simulink library "halout"  (R2021b)
settings: Solver=VariableStepAuto  StartTime=0.0  StopTime=10.0  RelTol=1e-3
undefined symbols (not defined in the file): C_TASK_5MS_S, FALSE, KHAL_CAN1FD1APS3E2E_flg, KHAL_CAN1FD1APS3TxReq_flg, KHAL_CAN1FD1VCU2E2E_flg, KHAL_CAN1FD1VCU2TxReq_flg, KHAL_CAN1FD1VCU3E2E_flg, KHAL_CAN1FD1VCU3TxReq_flg, KHAL_CAN1TxReq_flg, KHAL_CAN1VMCFCM1E2E_flg, KHAL_CAN1VMCFCM1TxReq_flg, KHAL_CAN2TxReq_flg, KHAL_CAN3FD3VCU1toNIDECTxReq_flg, KHAL_CAN3FD3VCU1TxReq_flg, KHAL_CAN3FD3VCU2E2E_flg, KHAL_CAN3FD3VCU2toNIDECE2E_flg, KHAL_CAN3FD3VCU2toNIDECTxReq_flg, KHAL_CAN3FD3VCU2TxReq_flg, KHAL_CAN3TxReq_flg, KHAL_CAN4FD4CE1000E2E_flg, KHAL_CAN4FD4CE1000TxReq_flg, KHAL_CAN4TxReq_flg, KHAL_CAN5TxReq_flg, KHAL_CAN6FD6APS3E2E_flg, KHAL_CAN6FD6APS3TxReq_flg, KHAL_CAN6FD6VCU2E2E_flg, KHAL_CAN6FD6VCU2TxReq_flg, KHAL_CAN6TxReq_flg, ONE_INT, TRUE, ZERO_INT
libraries: FVT_lib x549, simulink x244
(part 12 of 27)

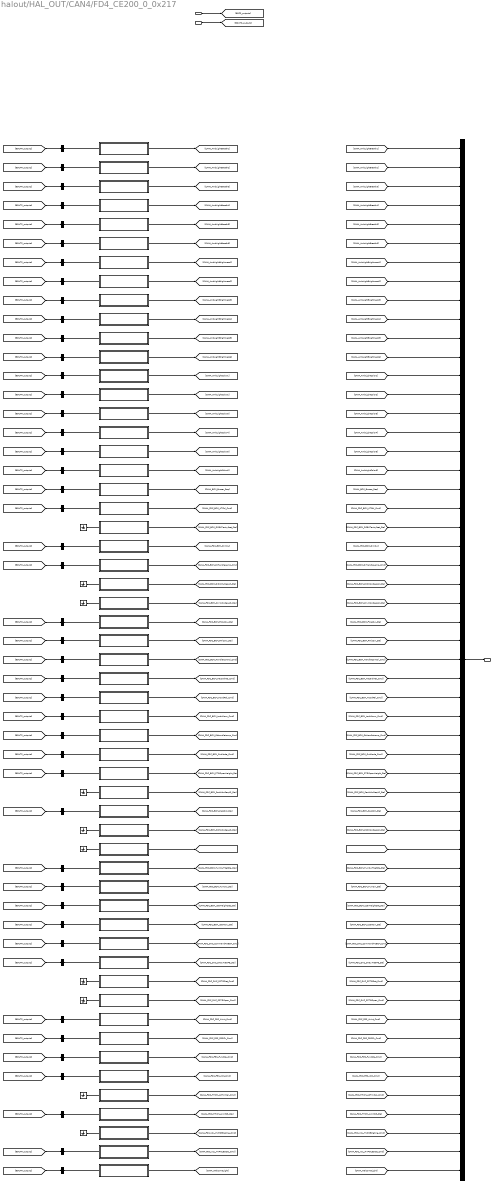
== system halout/HAL_OUT/CAN4/FD4_CE200_0_0x217 ==
  BSCP_outputs : Inport  OutDataTypeStr=Bus: BSCP_outputs
  BOUTP_outputs : Inport  Port=2  OutDataTypeStr=Bus: BOUTP_outputs
  AmbLightBreath1 : Subsystem
  AmbLightBreath2 : Subsystem
  AmbLightBreath3 : Subsystem
  AmbLightBreath4 : Subsystem
  AmbLightBreath5 : Subsystem
  AmbLightBreath6 : Subsystem
  AmbLightBrightness1 : Subsystem
  AmbLightBrightness2 : Subsystem
  AmbLightBrightness3 : Subsystem
  AmbLightBrightness4 : Subsystem
  AmbLightBrightness5 : Subsystem
  AmbLightBrightness6 : Subsystem
  AmbLightColor1 : Subsystem
  AmbLightColor2 : Subsystem
  AmbLightColor3 : Subsystem
  AmbLightColor4 : Subsystem
  AmbLightColor5 : Subsystem
  AmbLightColor6 : Subsystem
  BCMBuzzerReq : Subsystem
  FDCBCMATCtrlCmd : Subsystem
  FDCBCMDSEATentryfsetSta : Subsystem
  FDCBCMDimSw : Subsystem
  FDCBCMDrHandleLampCmd : Subsystem
  FDCBCMDrRWdwReqAPSta : Subsystem
  FDCBCMDrvWdwReqAPSta : Subsystem
  FDCBCMFWasSwSta : Subsystem
  FDCBCMFWipSwSta : Subsystem
  FDCBCMHandleControlCmd : Subsystem
  FDCBCMHazardINDCmd : Subsystem
  FDCBCMHoodRelCmd : Subsystem
  FDCBCMLockAlarmCmd : Subsystem
  FDCBCMOtHandleLampCmd : Subsystem
  FDCBCMOutModeCmd : Subsystem
  FDCBCMPTGOpenHeightSta : Subsystem
  FDCBCMPasWdwReqAPSta : Subsystem
  FDCBCMPassSWSta : Subsystem
  FDCBCMPsRWdwReqAPSta : Subsystem
  FDCBCMSettingUpdateReqCmd : Subsystem
  FDCBCMTurnSwSta : Subsystem
  FDCBCMTurnSwTSetStaSta : Subsystem
  FDCBCMUserHeightSetSta : Subsystem
  FDCBCMUserNowSta : Subsystem
  FDCDKCCommandToBCMCmd : Subsystem
  FDCDKCDKeyAreaPESta : Subsystem
  FDCDKCSPTGDetCmd : Subsystem
  FDCDKCSPTGOpenCmd : Subsystem
  FDCFGSAirIntCmd : Subsystem
  FDCFGSFGSChCmd : Subsystem
  FDCFGSFuncStaCmd : Subsystem
  FDCFGSIONCmd : Subsystem
  FDCTHCMACTInitialCmd : Subsystem
  FDCTHCMAirIntZ3Sta : Subsystem
  FDCV2LHVPOBklgtingCmd : Subsystem
  FDCV2LHVPOLEDStsCmd : Subsystem
  Ground{,2..3,6..12} (10 alike) : Ground
  WelcomeLight : Subsystem
  bus_creator : BusCreator  Inputs=55  OutDataTypeStr=Bus: DT_CAN4_SG_FD4_CE200_0  NonVirtualBus=on
  bus_selector : BusSelector  OutputSignals=VOUTP_AmbLightBreath1_enum
  bus_selector1 : BusSelector  OutputSignals=VOUTP_AmbLightBreath2_enum
  bus_selector10 : BusSelector  OutputSignals=VOUTP_AmbLightBrightness5_enum
  bus_selector11 : BusSelector  OutputSignals=VOUTP_AmbLightBrightness6_enum
  bus_selector12 : BusSelector  OutputSignals=VOUTP_AmbLightColor1_enum
  bus_selector13 : BusSelector  OutputSignals=VOUTP_AmbLightColor2_enum
  bus_selector14 : BusSelector  OutputSignals=VOUTP_AmbLightColor3_enum
  bus_selector15 : BusSelector  OutputSignals=VOUTP_AmbLightColor4_enum
  bus_selector16 : BusSelector  OutputSignals=VOUTP_AmbLightColor5_enum
  bus_selector17 : BusSelector  OutputSignals=VOUTP_AmbLightColor6_enum
  bus_selector18 : BusSelector  OutputSignals=VOUTP_BCMBuzzerReq_flg
  bus_selector19 : BusSelector  OutputSignals=VOUTP_ATCtrl_enum
  bus_selector2 : BusSelector  OutputSignals=VOUTP_AmbLightBreath3_enum
  bus_selector20 : BusSelector  OutputSignals=VOUTP_DimSwSta_flg
  bus_selector21 : BusSelector  OutputSignals=VOUTP_FWasSwSta_enum
  bus_selector22 : BusSelector  OutputSignals=VOUTP_FWipSwSta_enum
  bus_selector23 : BusSelector  OutputSignals=VOUTP_HazardIND_flg
  bus_selector24 : BusSelector  OutputSignals=VOUTP_HoodRelCmd_flg
  bus_selector25 : BusSelector  OutputSignals=VOUTP_LockAlarm_enum
  bus_selector26 : BusSelector  OutputSignals=VOUTP_OutMode_enum
  bus_selector27 : BusSelector  OutputSignals=VOUTP_PTGOpenHeightSta_enum
  bus_selector28 : BusSelector  OutputSignals=VOUTP_PassSWSta_flg
  bus_selector29 : BusSelector  OutputSignals=VOUTP_TurnSwTSetSta_enum
  bus_selector3 : BusSelector  OutputSignals=VOUTP_AmbLightBreath4_enum
  bus_selector30 : BusSelector  OutputSignals=VOUTP_TurnSwSta_enum
  bus_selector31 : BusSelector  OutputSignals=VOUTP_UserHeightSet_cnt
  bus_selector32 : BusSelector  OutputSignals=VOUTP_UserNow_enum
  bus_selector33 : BusSelector  OutputSignals=VOUTP_PCommandToBCM_enum
  bus_selector34 : BusSelector  OutputSignals=VOUTP_KeyAreaLockUnlock_enum
  bus_selector35 : BusSelector  OutputSignals=VOUTP_FDCFGSAirIntCmd_enum
  bus_selector36 : BusSelector  OutputSignals=VOUTP_FDCFGSChCmd_enum
  bus_selector37 : BusSelector  OutputSignals=VOUTP_FDCFGSFuncSta_flg
  bus_selector38 : BusSelector  OutputSignals=VOUTP_FDCFGSIONCmd_flg
  bus_selector39 : BusSelector  OutputSignals=VOUTP_FDCTHCAirIntZ3Sta_enum
  bus_selector4 : BusSelector  OutputSignals=VOUTP_AmbLightBreath5_enum
  bus_selector40 : BusSelector  OutputSignals=VOUTP_HVPO120VGrpALDSt_enum
  bus_selector41 : BusSelector  OutputSignals=VOUTP_WelcomeLight_enum
  bus_selector42 : BusSelector  OutputSignals=VOUTP_FDLHandleLampCmd_flg
  bus_selector43 : BusSelector  OutputSignals=VOUTP_FDHandleCmd_enum
  bus_selector44 : BusSelector  OutputSignals=VOUTP_FDRHandleLampCmd_flg
  bus_selector5 : BusSelector  OutputSignals=VOUTP_AmbLightBreath6_enum
  bus_selector6 : BusSelector  OutputSignals=VOUTP_AmbLightBrightness1_enum
  bus_selector7 : BusSelector  OutputSignals=VOUTP_AmbLightBrightness2_enum
  bus_selector8 : BusSelector  OutputSignals=VOUTP_AmbLightBrightness3_enum
  bus_selector9 : BusSelector  OutputSignals=VOUTP_AmbLightBrightness4_enum
  FD4_CE200_0 : Outport
  wires:
  BSCP_outputs/1 -> [BSCP_outputs]
  BOUTP_outputs/1 -> [BOUTP_outputs]
  [CAN4_AmbLightBreath1] -> bus_creator/1  "CAN4_AmbLightBreath1"
  [CAN4_AmbLightBreath2] -> bus_creator/2  "CAN4_AmbLightBreath2"
  [CAN4_AmbLightBreath3] -> bus_creator/3  "CAN4_AmbLightBreath3"
  [CAN4_AmbLightBreath4] -> bus_creator/4  "CAN4_AmbLightBreath4"
  [CAN4_AmbLightBreath5] -> bus_creator/5  "CAN4_AmbLightBreath5"
  [CAN4_AmbLightBreath6] -> bus_creator/6  "CAN4_AmbLightBreath6"
  [CAN4_AmbLightBrightness1] -> bus_creator/7  "CAN4_AmbLightBrightness1"
  [CAN4_AmbLightBrightness2] -> bus_creator/8  "CAN4_AmbLightBrightness2"
  [CAN4_AmbLightBrightness3] -> bus_creator/9  "CAN4_AmbLightBrightness3"
  [CAN4_AmbLightBrightness4] -> bus_creator/10  "CAN4_AmbLightBrightness4"
  [CAN4_AmbLightBrightness5] -> bus_creator/11  "CAN4_AmbLightBrightness5"
  [CAN4_AmbLightBrightness6] -> bus_creator/12  "CAN4_AmbLightBrightness6"
  [CAN4_AmbLightColor1] -> bus_creator/13  "CAN4_AmbLightColor1"
  [CAN4_AmbLightColor2] -> bus_creator/14  "CAN4_AmbLightColor2"
  [CAN4_AmbLightColor3] -> bus_creator/15  "CAN4_AmbLightColor3"
  [CAN4_AmbLightColor4] -> bus_creator/16  "CAN4_AmbLightColor4"
  [CAN4_AmbLightColor5] -> bus_creator/17  "CAN4_AmbLightColor5"
  [CAN4_AmbLightColor6] -> bus_creator/18  "CAN4_AmbLightColor6"
  [CAN4_BCM_Buzzer_Req] -> bus_creator/19  "CAN4_BCM_Buzzer_Req"
  [CAN4_FDC_BCM_ATCtrl_Cmd] -> bus_creator/20  "CAN4_FDC_BCM_ATCtrl_Cmd"
  [CAN4_FDC_BCM_DSEATentryfset_Sta] -> bus_creator/21  "CAN4_FDC_BCM_DSEATentryfset_Sta"
  [CAN4_FDC_BCM_DimSw] -> bus_creator/22  "CAN4_FDC_BCM_DimSw"
  [CAN4_FDC_BCM_DrHandleLamp_Cmd] -> bus_creator/23  "CAN4_FDC_BCM_DrHandleLamp_Cmd"
  [CAN4_FDC_BCM_DrRWdwReqAP_Sta] -> bus_creator/24  "CAN4_FDC_BCM_DrRWdwReqAP_Sta"
  [CAN4_FDC_BCM_DrvWdwReqAP_Sta] -> bus_creator/25  "CAN4_FDC_BCM_DrvWdwReqAP_Sta"
  [CAN4_FDC_BCM_FWasSw_Sta] -> bus_creator/26  "CAN4_FDC_BCM_FWasSw_Sta"
  [CAN4_FDC_BCM_FWipSw_Sta] -> bus_creator/27  "CAN4_FDC_BCM_FWipSw_Sta"
  [CAN4_FDC_BCM_HandleControl_Cmd] -> bus_creator/28  "CAN4_FDC_BCM_HandleControl_Cmd"
  [CAN4_FDC_BCM_HazardIND_Cmd] -> bus_creator/29  "CAN4_FDC_BCM_HazardIND_Cmd"
  [CAN4_FDC_BCM_HoodRel_Cmd] -> bus_creator/30  "CAN4_FDC_BCM_HoodRel_Cmd"
  [CAN4_FDC_BCM_LockAlarm_Cmd] -> bus_creator/31  "CAN4_FDC_BCM_LockAlarm_Cmd"
  [CAN4_FDC_BCM_OtHandleLamp_Cmd] -> bus_creator/32  "CAN4_FDC_BCM_OtHandleLamp_Cmd"
  [CAN4_FDC_BCM_OutMode_Cmd] -> bus_creator/33  "CAN4_FDC_BCM_OutMode_Cmd"
  [CAN4_FDC_BCM_PTGOpenHeight_Sta] -> bus_creator/34  "CAN4_FDC_BCM_PTGOpenHeight_Sta"
  [CAN4_FDC_BCM_PasWdwReqAP_Sta] -> bus_creator/35  "CAN4_FDC_BCM_PasWdwReqAP_Sta"
  [CAN4_FDC_BCM_PassSW_Sta] -> bus_creator/36  "CAN4_FDC_BCM_PassSW_Sta"
  [CAN4_FDC_BCM_PsRWdwReqAP_Sta] -> bus_creator/37  "CAN4_FDC_BCM_PsRWdwReqAP_Sta"
  [CAN4_FDC_BCM_SettingUpdateReq_Cmd] -> bus_creator/38  "CAN4_FDC_BCM_SettingUpdateReq_Cmd"
  [CAN4_FDC_BCM_TurnSwTSetSta_Sta] -> bus_creator/39  "CAN4_FDC_BCM_TurnSwTSetSta_Sta"
  [CAN4_FDC_BCM_TurnSw_Sta] -> bus_creator/40  "CAN4_FDC_BCM_TurnSw_Sta"
  [CAN4_FDC_BCM_UserHeightSet_Sta] -> bus_creator/41  "CAN4_FDC_BCM_UserHeightSet_Sta"
  [CAN4_FDC_BCM_UserNow_Sta] -> bus_creator/42  "CAN4_FDC_BCM_UserNow_Sta"
  [CAN4_FDC_DKC_CommandToBCM_Cmd] -> bus_creator/43  "CAN4_FDC_DKC_CommandToBCM_Cmd"
  [CAN4_FDC_DKC_DKeyAreaPE_Sta] -> bus_creator/44  "CAN4_FDC_DKC_DKeyAreaPE_Sta"
  [CAN4_FDC_DKC_SPTGDet_Cmd] -> bus_creator/45  "CAN4_FDC_DKC_SPTGDet_Cmd"
  [CAN4_FDC_DKC_SPTGOpen_Cmd] -> bus_creator/46  "CAN4_FDC_DKC_SPTGOpen_Cmd"
  [CAN4_FDC_FGS_AirInt_Cmd] -> bus_creator/47  "CAN4_FDC_FGS_AirInt_Cmd"
  [CAN4_FDC_FGS_FGSCh_Cmd] -> bus_creator/48  "CAN4_FDC_FGS_FGSCh_Cmd"
  [CAN4_FDC_FGS_FuncSta_Cmd] -> bus_creator/49  "CAN4_FDC_FGS_FuncSta_Cmd"
  [CAN4_FDC_FGS_ION_Cmd] -> bus_creator/50  "CAN4_FDC_FGS_ION_Cmd"
  [CAN4_FDC_THCM_ACTInitial_Cmd] -> bus_creator/51  "CAN4_FDC_THCM_ACTInitial_Cmd"
  [CAN4_FDC_THCM_AirIntZ3_Sta] -> bus_creator/52  "CAN4_FDC_THCM_AirIntZ3_Sta"
  [CAN4_FDC_V2L_HVPOBklgting_Cmd] -> bus_creator/53  "CAN4_FDC_V2L_HVPOBklgting_Cmd"
  [CAN4_FDC_V2L_HVPOLEDSts_Cmd] -> bus_creator/54  "CAN4_FDC_V2L_HVPOLEDSts_Cmd"
  [CAN4_WelcomeLight] -> bus_creator/55  "CAN4_WelcomeLight"
  bus_creator/1 -> FD4_CE200_0/1
  AmbLightBreath1/1(CAN4_AmbLightBreath1) -> [CAN4_AmbLightBreath1]
  AmbLightBreath2/1(CAN4_AmbLightBreath2) -> [CAN4_AmbLightBreath2]
  AmbLightBreath3/1(CAN4_AmbLightBreath3) -> [CAN4_AmbLightBreath3]
  AmbLightBreath4/1(CAN4_AmbLightBreath4) -> [CAN4_AmbLightBreath4]
  AmbLightBreath5/1(CAN4_AmbLightBreath5) -> [CAN4_AmbLightBreath5]
  AmbLightBreath6/1(CAN4_AmbLightBreath6) -> [CAN4_AmbLightBreath6]
  AmbLightBrightness1/1(CAN4_AmbLightBrightness1) -> [CAN4_AmbLightBrightness1]
  AmbLightBrightness2/1(CAN4_AmbLightBrightness2) -> [CAN4_AmbLightBrightness2]
  AmbLightBrightness3/1(CAN4_AmbLightBrightness3) -> [CAN4_AmbLightBrightness3]
  AmbLightBrightness4/1(CAN4_AmbLightBrightness4) -> [CAN4_AmbLightBrightness4]
  AmbLightBrightness5/1(CAN4_AmbLightBrightness5) -> [CAN4_AmbLightBrightness5]
  AmbLightBrightness6/1(CAN4_AmbLightBrightness6) -> [CAN4_AmbLightBrightness6]
  AmbLightColor1/1(CAN4_AmbLightColor1) -> [CAN4_AmbLightColor1]
  AmbLightColor2/1(CAN4_AmbLightColor2) -> [CAN4_AmbLightColor2]
  AmbLightColor3/1(CAN4_AmbLightColor3) -> [CAN4_AmbLightColor3]
  AmbLightColor4/1(CAN4_AmbLightColor4) -> [CAN4_AmbLightColor4]
  AmbLightColor5/1(CAN4_AmbLightColor5) -> [CAN4_AmbLightColor5]
  AmbLightColor6/1(CAN4_AmbLightColor6) -> [CAN4_AmbLightColor6]
  BCMBuzzerReq/1(CAN4_BCM_Buzzer_Req) -> [CAN4_BCM_Buzzer_Req]
  FDCBCMATCtrlCmd/1(CAN4_FDC_BCM_ATCtrl_Cmd) -> [CAN4_FDC_BCM_ATCtrl_Cmd]
  FDCBCMDSEATentryfsetSta/1(CAN4_FDC_BCM_DSEATentryfset_Sta) -> [CAN4_FDC_BCM_DSEATentryfset_Sta]
  FDCBCMDimSw/1(CAN4_FDC_BCM_DimSw) -> [CAN4_FDC_BCM_DimSw]
  FDCBCMDrHandleLampCmd/1(CAN4_FDC_BCM_DrHandleLamp_Cmd) -> [CAN4_FDC_BCM_DrHandleLamp_Cmd]
  FDCBCMDrRWdwReqAPSta/1(CAN4_FDC_BCM_DrRWdwReqAP_Sta) -> [CAN4_FDC_BCM_DrRWdwReqAP_Sta]
  FDCBCMDrvWdwReqAPSta/1(CAN4_FDC_BCM_DrvWdwReqAP_Sta) -> [CAN4_FDC_BCM_DrvWdwReqAP_Sta]
  FDCBCMFWasSwSta/1(CAN4_FDC_BCM_FWasSw_Sta) -> [CAN4_FDC_BCM_FWasSw_Sta]
  FDCBCMFWipSwSta/1(CAN4_FDC_BCM_FWipSw_Sta) -> [CAN4_FDC_BCM_FWipSw_Sta]
  FDCBCMHandleControlCmd/1(CAN4_FDC_BCM_HandleControl_Cmd) -> [CAN4_FDC_BCM_HandleControl_Cmd]
  FDCBCMHazardINDCmd/1(CAN4_FDC_BCM_HazardIND_Cmd) -> [CAN4_FDC_BCM_HazardIND_Cmd]
  FDCBCMHoodRelCmd/1(CAN4_FDC_BCM_HoodRel_Cmd) -> [CAN4_FDC_BCM_HoodRel_Cmd]
  FDCBCMLockAlarmCmd/1(CAN4_FDC_BCM_LockAlarm_Cmd) -> [CAN4_FDC_BCM_LockAlarm_Cmd]
  FDCBCMOtHandleLampCmd/1(CAN4_FDC_BCM_OtHandleLamp_Cmd) -> [CAN4_FDC_BCM_OtHandleLamp_Cmd]
  FDCBCMOutModeCmd/1(CAN4_FDC_BCM_OutMode_Cmd) -> [CAN4_FDC_BCM_OutMode_Cmd]
  FDCBCMPTGOpenHeightSta/1(CAN4_FDC_BCM_PTGOpenHeight_Sta) -> [CAN4_FDC_BCM_PTGOpenHeight_Sta]
  FDCBCMPasWdwReqAPSta/1(CAN4_FDC_BCM_PasWdwReqAP_Sta) -> [CAN4_FDC_BCM_PasWdwReqAP_Sta]
  FDCBCMPassSWSta/1(CAN4_FDC_BCM_PassSW_Sta) -> [CAN4_FDC_BCM_PassSW_Sta]
  FDCBCMPsRWdwReqAPSta/1(CAN4_FDC_BCM_PsRWdwReqAP_Sta) -> [CAN4_FDC_BCM_PsRWdwReqAP_Sta]
  FDCBCMSettingUpdateReqCmd/1(CAN4_FDC_BCM_SettingUpdateReq_Cmd) -> [CAN4_FDC_BCM_SettingUpdateReq_Cmd]
  FDCBCMTurnSwTSetStaSta/1(CAN4_FDC_BCM_TurnSwTSetSta_Sta) -> [CAN4_FDC_BCM_TurnSwTSetSta_Sta]
  FDCBCMTurnSwSta/1(CAN4_FDC_BCM_TurnSw_Sta) -> [CAN4_FDC_BCM_TurnSw_Sta]
  FDCBCMUserHeightSetSta/1(CAN4_FDC_BCM_UserHeightSet_Sta) -> [CAN4_FDC_BCM_UserHeightSet_Sta]
  FDCBCMUserNowSta/1(CAN4_FDC_BCM_UserNow_Sta) -> [CAN4_FDC_BCM_UserNow_Sta]
  FDCDKCCommandToBCMCmd/1(CAN4_FDC_DKC_CommandToBCM_Cmd) -> [CAN4_FDC_DKC_CommandToBCM_Cmd]
  FDCDKCDKeyAreaPESta/1(CAN4_FDC_DKC_DKeyAreaPE_Sta) -> [CAN4_FDC_DKC_DKeyAreaPE_Sta]
  FDCDKCSPTGDetCmd/1(CAN4_FDC_DKC_SPTGDet_Cmd) -> [CAN4_FDC_DKC_SPTGDet_Cmd]
  FDCDKCSPTGOpenCmd/1(CAN4_FDC_DKC_SPTGOpen_Cmd) -> [CAN4_FDC_DKC_SPTGOpen_Cmd]
  FDCFGSAirIntCmd/1(CAN4_FDC_FGS_AirInt_Cmd) -> [CAN4_FDC_FGS_AirInt_Cmd]
  FDCFGSFGSChCmd/1(CAN4_FDC_FGS_FGSCh_Cmd) -> [CAN4_FDC_FGS_FGSCh_Cmd]
  FDCFGSFuncStaCmd/1(CAN4_FDC_FGS_FuncSta_Cmd) -> [CAN4_FDC_FGS_FuncSta_Cmd]
  FDCFGSIONCmd/1(CAN4_FDC_FGS_ION_Cmd) -> [CAN4_FDC_FGS_ION_Cmd]
  FDCTHCMACTInitialCmd/1(CAN4_FDC_THCM_ACTInitial_Cmd) -> [CAN4_FDC_THCM_ACTInitial_Cmd]
  FDCTHCMAirIntZ3Sta/1(CAN4_FDC_THCM_AirIntZ3_Sta) -> [CAN4_FDC_THCM_AirIntZ3_Sta]
  FDCV2LHVPOBklgtingCmd/1(CAN4_FDC_V2L_HVPOBklgting_Cmd) -> [CAN4_FDC_V2L_HVPOBklgting_Cmd]
  FDCV2LHVPOLEDStsCmd/1(CAN4_FDC_V2L_HVPOLEDSts_Cmd) -> [CAN4_FDC_V2L_HVPOLEDSts_Cmd]
  WelcomeLight/1(CAN4_WelcomeLight) -> [CAN4_WelcomeLight]
  bus_selector/1 -> AmbLightBreath1/1(AmbLightBreath1)  "<VOUTP_AmbLightBreath1_enum>"
  [BOUTP_outputs] -> bus_selector/1
  bus_selector1/1 -> AmbLightBreath2/1(AmbLightBreath2)  "<VOUTP_AmbLightBreath2_enum>"
  [BOUTP_outputs] -> bus_selector1/1
  bus_selector2/1 -> AmbLightBreath3/1(AmbLightBreath3)  "<VOUTP_AmbLightBreath3_enum>"
  [BOUTP_outputs] -> bus_selector2/1
  bus_selector3/1 -> AmbLightBreath4/1(AmbLightBreath4)  "<VOUTP_AmbLightBreath4_enum>"
  [BOUTP_outputs] -> bus_selector3/1
  bus_selector4/1 -> AmbLightBreath5/1(AmbLightBreath5)  "<VOUTP_AmbLightBreath5_enum>"
  [BOUTP_outputs] -> bus_selector4/1
  bus_selector5/1 -> AmbLightBreath6/1(AmbLightBreath6)  "<VOUTP_AmbLightBreath6_enum>"
  [BOUTP_outputs] -> bus_selector5/1
  bus_selector6/1 -> AmbLightBrightness1/1(AmbLightBrightness1)  "<VOUTP_AmbLightBrightness1_enum>"
  [BOUTP_outputs] -> bus_selector6/1
  bus_selector7/1 -> AmbLightBrightness2/1(AmbLightBrightness2)  "<VOUTP_AmbLightBrightness2_enum>"
  [BOUTP_outputs] -> bus_selector7/1
  bus_selector8/1 -> AmbLightBrightness3/1(AmbLightBrightness3)  "<VOUTP_AmbLightBrightness3_enum>"
  [BOUTP_outputs] -> bus_selector8/1
  bus_selector9/1 -> AmbLightBrightness4/1(AmbLightBrightness4)  "<VOUTP_AmbLightBrightness4_enum>"
  [BOUTP_outputs] -> bus_selector9/1
  bus_selector10/1 -> AmbLightBrightness5/1(AmbLightBrightness5)  "<VOUTP_AmbLightBrightness5_enum>"
  [BOUTP_outputs] -> bus_selector10/1
  bus_selector11/1 -> AmbLightBrightness6/1(AmbLightBrightness6)  "<VOUTP_AmbLightBrightness6_enum>"
  [BOUTP_outputs] -> bus_selector11/1
  bus_selector12/1 -> AmbLightColor1/1(AmbLightColor1)  "<VOUTP_AmbLightColor1_enum>"
  [BOUTP_outputs] -> bus_selector12/1
  bus_selector13/1 -> AmbLightColor2/1(AmbLightColor2)  "<VOUTP_AmbLightColor2_enum>"
  [BOUTP_outputs] -> bus_selector13/1
  bus_selector14/1 -> AmbLightColor3/1(AmbLightColor3)  "<VOUTP_AmbLightColor3_enum>"
  [BOUTP_outputs] -> bus_selector14/1
  bus_selector15/1 -> AmbLightColor4/1(AmbLightColor4)  "<VOUTP_AmbLightColor4_enum>"
  [BOUTP_outputs] -> bus_selector15/1
  bus_selector16/1 -> AmbLightColor5/1(AmbLightColor5)  "<VOUTP_AmbLightColor5_enum>"
  [BOUTP_outputs] -> bus_selector16/1
  bus_selector17/1 -> AmbLightColor6/1(AmbLightColor6)  "<VOUTP_AmbLightColor6_enum>"
  [BOUTP_outputs] -> bus_selector17/1
  bus_selector18/1 -> BCMBuzzerReq/1(BCMBuzzerReq)  "<VOUTP_BCMBuzzerReq_flg>"
  [BOUTP_outputs] -> bus_selector18/1
  bus_selector19/1 -> FDCBCMATCtrlCmd/1(FDCBCMATCtrlCmd)  "<VOUTP_ATCtrl_enum>"
  [BOUTP_outputs] -> bus_selector19/1
  Ground/1 -> FDCBCMDSEATentryfsetSta/1(FDCBCMDSEATentryfsetSta)
  bus_selector20/1 -> FDCBCMDimSw/1(FDCBCMDimSw)  "<VOUTP_DimSwSta_flg>"
  [BOUTP_outputs] -> bus_selector20/1
  Ground2/1 -> FDCBCMDrRWdwReqAPSta/1(FDCBCMDrRWdwReqAPSta)
  Ground3/1 -> FDCBCMDrvWdwReqAPSta/1(FDCBCMDrvWdwReqAPSta)
  bus_selector21/1 -> FDCBCMFWasSwSta/1(FDCBCMFWasSwSta)  "<VOUTP_FWasSwSta_enum>"
  [BOUTP_outputs] -> bus_selector21/1
  bus_selector22/1 -> FDCBCMFWipSwSta/1(FDCBCMFWipSwSta)  "<VOUTP_FWipSwSta_enum>"
  [BOUTP_outputs] -> bus_selector22/1
  bus_selector23/1 -> FDCBCMHazardINDCmd/1(FDCBCMHazardINDCmd)  "<VOUTP_HazardIND_flg>"
  [BOUTP_outputs] -> bus_selector23/1
  bus_selector24/1 -> FDCBCMHoodRelCmd/1(FDCBCMHoodRelCmd)  "<VOUTP_HoodRelCmd_flg>"
  [BOUTP_outputs] -> bus_selector24/1
  bus_selector25/1 -> FDCBCMLockAlarmCmd/1(FDCBCMLockAlarmCmd)  "<VOUTP_LockAlarm_enum>"
  [BOUTP_outputs] -> bus_selector25/1
  bus_selector26/1 -> FDCBCMOutModeCmd/1(FDCBCMOutModeCmd)  "<VOUTP_OutMode_enum>"
  [BOUTP_outputs] -> bus_selector26/1
  bus_selector27/1 -> FDCBCMPTGOpenHeightSta/1(FDCBCMPTGOpenHeightSta)  "<VOUTP_PTGOpenHeightSta_enum>"
  [BOUTP_outputs] -> bus_selector27/1
  Ground6/1 -> FDCBCMPasWdwReqAPSta/1(FDCBCMPasWdwReqAPSta)
  bus_selector28/1 -> FDCBCMPassSWSta/1(FDCBCMPassSWSta)  "<VOUTP_PassSWSta_flg>"
  [BOUTP_outputs] -> bus_selector28/1
  Ground7/1 -> FDCBCMPsRWdwReqAPSta/1(FDCBCMPsRWdwReqAPSta)
  Ground8/1 -> FDCBCMSettingUpdateReqCmd/1(FDCBCMSettingUpdateReqCmd)
  bus_selector29/1 -> FDCBCMTurnSwTSetStaSta/1(FDCBCMTurnSwTSetStaSta)  "<VOUTP_TurnSwTSetSta_enum>"
  [BOUTP_outputs] -> bus_selector29/1
  bus_selector30/1 -> FDCBCMTurnSwSta/1(FDCBCMTurnSwSta)  "<VOUTP_TurnSwSta_enum>"
  [BOUTP_outputs] -> bus_selector30/1
  bus_selector31/1 -> FDCBCMUserHeightSetSta/1(FDCBCMUserHeightSetSta)  "<VOUTP_UserHeightSet_cnt>"
  [BOUTP_outputs] -> bus_selector31/1
  bus_selector32/1 -> FDCBCMUserNowSta/1(FDCBCMUserNowSta)  "<VOUTP_UserNow_enum>"
  [BOUTP_outputs] -> bus_selector32/1
  bus_selector33/1 -> FDCDKCCommandToBCMCmd/1(FDCDKCCommandToBCMCmd)  "<VOUTP_PCommandToBCM_enum>"
  [BOUTP_outputs] -> bus_selector33/1
  bus_selector34/1 -> FDCDKCDKeyAreaPESta/1(FDCDKCDKeyAreaPESta)  "<VOUTP_KeyAreaLockUnlock_enum>"
  [BOUTP_outputs] -> bus_selector34/1
  Ground9/1 -> FDCDKCSPTGDetCmd/1(FDCDKCSPTGDetCmd)
  Ground10/1 -> FDCDKCSPTGOpenCmd/1(FDCDKCSPTGOpenCmd)
  bus_selector35/1 -> FDCFGSAirIntCmd/1(FDCFGSAirIntCmd)  "<VOUTP_FDCFGSAirIntCmd_enum>"
  [BOUTP_outputs] -> bus_selector35/1
  bus_selector36/1 -> FDCFGSFGSChCmd/1(FDCFGSFGSChCmd)  "<VOUTP_FDCFGSChCmd_enum>"
  [BOUTP_outputs] -> bus_selector36/1
  bus_selector37/1 -> FDCFGSFuncStaCmd/1(FDCFGSFuncStaCmd)  "<VOUTP_FDCFGSFuncSta_flg>"
  [BOUTP_outputs] -> bus_selector37/1
  bus_selector38/1 -> FDCFGSIONCmd/1(FDCFGSIONCmd)  "<VOUTP_FDCFGSIONCmd_flg>"
  [BOUTP_outputs] -> bus_selector38/1
  Ground11/1 -> FDCTHCMACTInitialCmd/1(FDCTHCMACTInitialCmd)
  bus_selector39/1 -> FDCTHCMAirIntZ3Sta/1(FDCTHCMAirIntZ3Sta)  "<VOUTP_FDCTHCAirIntZ3Sta_enum>"
  [BOUTP_outputs] -> bus_selector39/1
  Ground12/1 -> FDCV2LHVPOBklgtingCmd/1(FDCV2LHVPOBklgtingCmd)
  bus_selector40/1 -> FDCV2LHVPOLEDStsCmd/1(FDCV2LHVPOLEDStsCmd)  "<VOUTP_HVPO120VGrpALDSt_enum>"
  [BOUTP_outputs] -> bus_selector40/1
  bus_selector41/1 -> WelcomeLight/1(WelcomeLight)  "<VOUTP_WelcomeLight_enum>"
  [BOUTP_outputs] -> bus_selector41/1
  bus_selector42/1 -> FDCBCMDrHandleLampCmd/1(FDCBCMDrHandleLampCmd)  "<VOUTP_FDLHandleLampCmd_flg>"
  [BOUTP_outputs] -> bus_selector42/1
  bus_selector43/1 -> FDCBCMHandleControlCmd/1(FDCBCMHandleControlCmd)  "<VOUTP_FDHandleCmd_enum>"
  [BOUTP_outputs] -> bus_selector43/1
  [BOUTP_outputs] -> bus_selector44/1
  bus_selector44/1 -> FDCBCMOtHandleLampCmd/1(FDCBCMOtHandleLampCmd)  "<VOUTP_FDRHandleLampCmd_flg>"

== system halout/HAL_OUT/CAN4/Function-Call Subsystem ==
  function : TriggerPort  TriggerType=function-call  VariantControl=(inherit)
  Add : Sum
  Constant : Constant  Value=ONE_INT
  Constant1 : Constant  Value=ZERO_INT
  Constant2 : Constant  Value=uint8(10)
  GreaterThan : RelationalOperator  Operator=>  OutDataTypeStr=boolean  RndMeth=Simplest
  Switch : Switch  Criteria=u2 ~= 0
  Unit Delay : UnitDelay  SampleTime=-1  HasFrameUpgradeWarning=on
  TriggerCAN4VCU1_CNT : Outport
  wires:
  Add/1 -> Switch/3, GreaterThan/1
  Unit Delay/1 -> Add/1
  Constant/1 -> Add/2
  Switch/1 -> TriggerCAN4VCU1_CNT/1, Unit Delay/1
  Constant2/1 -> GreaterThan/2
  GreaterThan/1 -> Switch/2
  Constant1/1 -> Switch/1

== system halout/HAL_OUT/CAN4/GW4_CE100_0_0x253 ==
  BSCP_outputs : Inport  OutDataTypeStr=Bus: BSCP_outputs
  BOUTP_outputs : Inport  Port=2  OutDataTypeStr=Bus: BOUTP_outputs
  FDCBCMDrRWdwCtrlCmd : Subsystem
  FDCBCMDrvWdwCtrlCmd : Subsystem
  FDCBCMPasWdwCtrlCmd : Subsystem
  FDCBCMPsRWdwCtrlCmd : Subsystem
  FDCBCMSenstivityPosnCmd : Subsystem
  FDCPTGinnerSW2 : Subsystem
  bus_creator : BusCreator  Inputs=6  OutDataTypeStr=Bus: DT_CAN4_SG_GW4_CE100_0  NonVirtualBus=on
  bus_selector : BusSelector  OutputSignals=VOUTP_DrvWdwCtrlCmd_pct
  bus_selector1 : BusSelector  OutputSignals=VOUTP_PasWdwCtrlCmd_pct
  bus_selector2 : BusSelector  OutputSignals=VOUTP_SenstivityPosnCmd_enum
  bus_selector3 : BusSelector  OutputSignals=VOUTP_PTGInnerSW2_enum
  bus_selector4 : BusSelector  OutputSignals=VOUTP_DrRWdwCtrlCmd_pct
  bus_selector5 : BusSelector  OutputSignals=VOUTP_PsRWdwCtrlCmd_pct
  GW4_CE100_0 : Outport
  wires:
  BSCP_outputs/1 -> [BSCP_outputs]
  BOUTP_outputs/1 -> [BOUTP_outputs]
  [CAN4_FDC_BCM_DrRWdwCtrl_Cmd] -> bus_creator/1  "CAN4_FDC_BCM_DrRWdwCtrl_Cmd"
  [CAN4_FDC_BCM_DrvWdwCtrl_Cmd] -> bus_creator/2  "CAN4_FDC_BCM_DrvWdwCtrl_Cmd"
  [CAN4_FDC_BCM_PasWdwCtrl_Cmd] -> bus_creator/3  "CAN4_FDC_BCM_PasWdwCtrl_Cmd"
  [CAN4_FDC_BCM_PsRWdwCtrl_Cmd] -> bus_creator/4  "CAN4_FDC_BCM_PsRWdwCtrl_Cmd"
  [CAN4_FDC_BCM_SenstivityPosn_Cmd] -> bus_creator/5  "CAN4_FDC_BCM_SenstivityPosn_Cmd"
  [CAN4_FDC_PTG_inner_SW_2] -> bus_creator/6  "CAN4_FDC_PTG_inner_SW_2"
  bus_creator/1 -> GW4_CE100_0/1
  FDCBCMDrRWdwCtrlCmd/1(CAN4_FDC_BCM_DrRWdwCtrl_Cmd) -> [CAN4_FDC_BCM_DrRWdwCtrl_Cmd]
  FDCBCMDrvWdwCtrlCmd/1(CAN4_FDC_BCM_DrvWdwCtrl_Cmd) -> [CAN4_FDC_BCM_DrvWdwCtrl_Cmd]
  FDCBCMPasWdwCtrlCmd/1(CAN4_FDC_BCM_PasWdwCtrl_Cmd) -> [CAN4_FDC_BCM_PasWdwCtrl_Cmd]
  FDCBCMPsRWdwCtrlCmd/1(CAN4_FDC_BCM_PsRWdwCtrl_Cmd) -> [CAN4_FDC_BCM_PsRWdwCtrl_Cmd]
  FDCBCMSenstivityPosnCmd/1(CAN4_FDC_BCM_SenstivityPosn_Cmd) -> [CAN4_FDC_BCM_SenstivityPosn_Cmd]
  FDCPTGinnerSW2/1(CAN4_FDC_PTG_inner_SW_2) -> [CAN4_FDC_PTG_inner_SW_2]
  bus_selector/1 -> FDCBCMDrvWdwCtrlCmd/1(FDCBCMDrvWdwCtrlCmd)  "<VOUTP_DrvWdwCtrlCmd_pct>"
  [BOUTP_outputs] -> bus_selector/1
  bus_selector1/1 -> FDCBCMPasWdwCtrlCmd/1(FDCBCMPasWdwCtrlCmd)  "<VOUTP_PasWdwCtrlCmd_pct>"
  [BOUTP_outputs] -> bus_selector1/1
  bus_selector2/1 -> FDCBCMSenstivityPosnCmd/1(FDCBCMSenstivityPosnCmd)  "<VOUTP_SenstivityPosnCmd_enum>"
  [BOUTP_outputs] -> bus_selector2/1
  bus_selector3/1 -> FDCPTGinnerSW2/1(FDCPTGinnerSW2)  "<VOUTP_PTGInnerSW2_enum>"
  [BOUTP_outputs] -> bus_selector3/1
  bus_selector4/1 -> FDCBCMDrRWdwCtrlCmd/1(FDCBCMDrRWdwCtrlCmd)  "<VOUTP_DrRWdwCtrlCmd_pct>"
  [BOUTP_outputs] -> bus_selector4/1
  bus_selector5/1 -> FDCBCMPsRWdwCtrlCmd/1(FDCBCMPsRWdwCtrlCmd)  "<VOUTP_PsRWdwCtrlCmd_pct>"
  [BOUTP_outputs] -> bus_selector5/1

== system halout/HAL_OUT/CAN5/FD5_CE100_0_0x118 ==
  BSCP_outputs : Inport  OutDataTypeStr=Bus: BSCP_outputs
  BOUTP_outputs : Inport  Port=2  OutDataTypeStr=Bus: BOUTP_outputs
  AllDoorSW : Subsystem
  AntitheftSta : Subsystem
  BCMDoorLockSta : Subsystem
  CCUACLampSts : Subsystem
  CCUCbnPreACWkSts : Subsystem
  CCUCbnPreEstimdTi : Subsystem
  CCUCbnPreSts : Subsystem
  FDTBOXDTCDataErr : Subsystem
  FDTBOXDTCDataSta : Subsystem
  FDTBOXVehDataErr : Subsystem
  FDTBOXVehDataSta : Subsystem
  Ground{,1..6} (7 alike) : Ground
  HoodSW : Subsystem
  LowSOCWarn : Subsystem
  PwrSta : Subsystem
  ReVehThdChkSta : Subsystem
  ShiftGearPosn : Subsystem
  TCountSta : Subsystem
  TailgateRemote : Subsystem
  TailgateSW : Subsystem
  VehMalfunLevel : Subsystem
  bus_creator : BusCreator  Inputs=20  OutDataTypeStr=Bus: DT_CAN5_SG_FD5_CE100_0  NonVirtualBus=on
  bus_selector : BusSelector  OutputSignals=VOUTP_AllDoorSW_flg
  bus_selector1 : BusSelector  OutputSignals=VOUTP_AntitheftSta_enum
  bus_selector10 : BusSelector  OutputSignals=VOUTP_TailgateRemote_enum
  bus_selector11 : BusSelector  OutputSignals=VOUTP_TailgateSW_flg
  bus_selector12 : BusSelector  OutputSignals=VOUTP_VehMalfunLevel_enum
  bus_selector2 : BusSelector  OutputSignals=VOUTP_BCMDoorLockSta_flg
  bus_selector3 : BusSelector  OutputSignals=VOUTP_CCUACLampSts_flg
  bus_selector4 : BusSelector  OutputSignals=VOUTP_HoodSW_flg
  bus_selector5 : BusSelector  OutputSignals=VOUTP_LowSOCWarn_enum
  bus_selector6 : BusSelector  OutputSignals=VOUTP_PowerSta_enum
  bus_selector7 : BusSelector  OutputSignals=VOUTP_ReVehThdChkSta_enum
  bus_selector8 : BusSelector  OutputSignals=VOUTP_ShiftGearPosn_enum
  bus_selector9 : BusSelector  OutputSignals=VOUTP_TCountSta_enum
  FD5_CE100_0 : Outport
  wires:
  BSCP_outputs/1 -> [BSCP_outputs]
  BOUTP_outputs/1 -> [BOUTP_outputs]
  [CAN5_AllDoorSW] -> bus_creator/1  "CAN5_AllDoorSW"
  [CAN5_AntitheftSta] -> bus_creator/2  "CAN5_AntitheftSta"
  [CAN5_BCM_DoorLock_Sta] -> bus_creator/3  "CAN5_BCM_DoorLock_Sta"
  [CAN5_CCU_ACLampSts] -> bus_creator/4  "CAN5_CCU_ACLampSts"
  [CAN5_CCU_CbnPreACWkSts] -> bus_creator/5  "CAN5_CCU_CbnPreACWkSts"
  [CAN5_CCU_CbnPreEstimdTi] -> bus_creator/6  "CAN5_CCU_CbnPreEstimdTi"
  [CAN5_CCU_CbnPreSts] -> bus_creator/7  "CAN5_CCU_CbnPreSts"
  [CAN5_FD_TBOX_DTCData_Err] -> bus_creator/8  "CAN5_FD_TBOX_DTCData_Err"
  [CAN5_FD_TBOX_DTCData_Sta] -> bus_creator/9  "CAN5_FD_TBOX_DTCData_Sta"
  [CAN5_FD_TBOX_VehData_Err] -> bus_creator/10  "CAN5_FD_TBOX_VehData_Err"
  [CAN5_FD_TBOX_VehData_Sta] -> bus_creator/11  "CAN5_FD_TBOX_VehData_Sta"
  [CAN5_HoodSW] -> bus_creator/12  "CAN5_HoodSW"
  [CAN5_LowSOCWarn] -> bus_creator/13  "CAN5_LowSOCWarn"
  [CAN5_PwrSta] -> bus_creator/14  "CAN5_PwrSta"
  [CAN5_Re_VehThdChkSta] -> bus_creator/15  "CAN5_Re_VehThdChkSta"
  [CAN5_ShiftGearPosn] -> bus_creator/16  "CAN5_ShiftGearPosn"
  [CAN5_TCountSta] -> bus_creator/17  "CAN5_TCountSta"
  [CAN5_TailgateRemote] -> bus_creator/18  "CAN5_TailgateRemote"
  [CAN5_Tailgate_SW] -> bus_creator/19  "CAN5_Tailgate_SW"
  [CAN5_VehMalfunLevel] -> bus_creator/20  "CAN5_VehMalfunLevel"
  bus_creator/1 -> FD5_CE100_0/1
  AllDoorSW/1(CAN5_AllDoorSW) -> [CAN5_AllDoorSW]
  AntitheftSta/1(CAN5_AntitheftSta) -> [CAN5_AntitheftSta]
  BCMDoorLockSta/1(CAN5_BCM_DoorLock_Sta) -> [CAN5_BCM_DoorLock_Sta]
  CCUACLampSts/1(CAN5_CCU_ACLampSts) -> [CAN5_CCU_ACLampSts]
  CCUCbnPreACWkSts/1(CAN5_CCU_CbnPreACWkSts) -> [CAN5_CCU_CbnPreACWkSts]
  CCUCbnPreEstimdTi/1(CAN5_CCU_CbnPreEstimdTi) -> [CAN5_CCU_CbnPreEstimdTi]
  CCUCbnPreSts/1(CAN5_CCU_CbnPreSts) -> [CAN5_CCU_CbnPreSts]
  FDTBOXDTCDataErr/1(CAN5_FD_TBOX_DTCData_Err) -> [CAN5_FD_TBOX_DTCData_Err]
  FDTBOXDTCDataSta/1(CAN5_FD_TBOX_DTCData_Sta) -> [CAN5_FD_TBOX_DTCData_Sta]
  FDTBOXVehDataErr/1(CAN5_FD_TBOX_VehData_Err) -> [CAN5_FD_TBOX_VehData_Err]
  FDTBOXVehDataSta/1(CAN5_FD_TBOX_VehData_Sta) -> [CAN5_FD_TBOX_VehData_Sta]
  HoodSW/1(CAN5_HoodSW) -> [CAN5_HoodSW]
  LowSOCWarn/1(CAN5_LowSOCWarn) -> [CAN5_LowSOCWarn]
  PwrSta/1(CAN5_PwrSta) -> [CAN5_PwrSta]
  ReVehThdChkSta/1(CAN5_Re_VehThdChkSta) -> [CAN5_Re_VehThdChkSta]
  ShiftGearPosn/1(CAN5_ShiftGearPosn) -> [CAN5_ShiftGearPosn]
  TCountSta/1(CAN5_TCountSta) -> [CAN5_TCountSta]
  TailgateRemote/1(CAN5_TailgateRemote) -> [CAN5_TailgateRemote]
  TailgateSW/1(CAN5_Tailgate_SW) -> [CAN5_Tailgate_SW]
  VehMalfunLevel/1(CAN5_VehMalfunLevel) -> [CAN5_VehMalfunLevel]
  bus_selector/1 -> AllDoorSW/1(AllDoorSW)  "<VOUTP_AllDoorSW_flg>"
  [BOUTP_outputs] -> bus_selector/1
  bus_selector1/1 -> AntitheftSta/1(AntitheftSta)  "<VOUTP_AntitheftSta_enum>"
  [BOUTP_outputs] -> bus_selector1/1
  bus_selector2/1 -> BCMDoorLockSta/1(BCMDoorLockSta)  "<VOUTP_BCMDoorLockSta_flg>"
  [BOUTP_outputs] -> bus_selector2/1
  bus_selector3/1 -> CCUACLampSts/1(CCUACLampSts)  "<VOUTP_CCUACLampSts_flg>"
  [BOUTP_outputs] -> bus_selector3/1
  Ground/1 -> CCUCbnPreACWkSts/1(CCUCbnPreACWkSts)
  Ground1/1 -> CCUCbnPreEstimdTi/1(CCUCbnPreEstimdTi)
  Ground2/1 -> CCUCbnPreSts/1(CCUCbnPreSts)
  Ground3/1 -> FDTBOXDTCDataErr/1(FDTBOXDTCDataErr)
  Ground4/1 -> FDTBOXDTCDataSta/1(FDTBOXDTCDataSta)
  Ground5/1 -> FDTBOXVehDataErr/1(FDTBOXVehDataErr)
  Ground6/1 -> FDTBOXVehDataSta/1(FDTBOXVehDataSta)
  bus_selector4/1 -> HoodSW/1(HoodSW)  "<VOUTP_HoodSW_flg>"
  [BOUTP_outputs] -> bus_selector4/1
  bus_selector5/1 -> LowSOCWarn/1(LowSOCWarn)  "<VOUTP_LowSOCWarn_enum>"
  [BOUTP_outputs] -> bus_selector5/1
  bus_selector6/1 -> PwrSta/1(PwrSta)  "<VOUTP_PowerSta_enum>"
  [BOUTP_outputs] -> bus_selector6/1
  bus_selector7/1 -> ReVehThdChkSta/1(ReVehThdChkSta)  "<VOUTP_ReVehThdChkSta_enum>"
  [BOUTP_outputs] -> bus_selector7/1
  bus_selector8/1 -> ShiftGearPosn/1(ShiftGearPosn)  "<VOUTP_ShiftGearPosn_enum>"
  [BOUTP_outputs] -> bus_selector8/1
  bus_selector9/1 -> TCountSta/1(TCountSta)  "<VOUTP_TCountSta_enum>"
  [BOUTP_outputs] -> bus_selector9/1
  bus_selector10/1 -> TailgateRemote/1(TailgateRemote)  "<VOUTP_TailgateRemote_enum>"
  [BOUTP_outputs] -> bus_selector10/1
  bus_selector11/1 -> TailgateSW/1(TailgateSW)  "<VOUTP_TailgateSW_flg>"
  [BOUTP_outputs] -> bus_selector11/1
  bus_selector12/1 -> VehMalfunLevel/1(VehMalfunLevel)  "<VOUTP_VehMalfunLevel_enum>"
  [BOUTP_outputs] -> bus_selector12/1

== system halout/HAL_OUT/CAN5/FD5_Debug1_0x4D0 ==
  BSCP_outputs : Inport  OutDataTypeStr=Bus: BSCP_outputs
  BOUTP_outputs : Inport  Port=2  OutDataTypeStr=Bus: BOUTP_outputs
  ID1ALTU : Subsystem
  ID1LocALTU : Subsystem
  ID1messageALTU : Subsystem
  ID2ALTU : Subsystem
  ID2LocALTU : Subsystem
  ID2messageALTU : Subsystem
  ID3ALTU : Subsystem
  ID3LocALTU : Subsystem
  ID3messageALTU : Subsystem
  ID4ALTU : Subsystem
  ID4LocALTU : Subsystem
  ID4messageALTU : Subsystem
  IDinALTU : Subsystem
  LFSensorMode : Subsystem
  LRSensorMode : Subsystem
  RFFATALTU : Subsystem
  RFSensorMode : Subsystem
  RRSensorMode : Subsystem
  S1WheelDebugALTU : Subsystem
  S2WheelDebugALTU : Subsystem
  S3WheelDebugALTU : Subsystem
  S4WheelDebugALTU : Subsystem
  bus_creator : BusCreator  Inputs=22  OutDataTypeStr=Bus: DT_CAN5_SG_FD5_Debug1  NonVirtualBus=on
  bus_selector : BusSelector  OutputSignals=VOUTP_S1ID_raw32
  bus_selector1 : BusSelector  OutputSignals=VOUTP_S1L_enum
  bus_selector10 : BusSelector  OutputSignals=VOUTP_S4L_enum
  bus_selector11 : BusSelector  OutputSignals=VOUTP_ID4messageALTU_raw8
  bus_selector12 : BusSelector  OutputSignals=VOUTP_IDin_raw32
  bus_selector13 : BusSelector  OutputSignals=VOUTP_LFSensorMode_flg
  bus_selector14 : BusSelector  OutputSignals=VOUTP_LRSensorMode_flg
  bus_selector15 : BusSelector  OutputSignals=VOUTP_RFSensorMode_flg
  bus_selector16 : BusSelector  OutputSignals=VOUTP_FAT_flg
  bus_selector17 : BusSelector  OutputSignals=VOUTP_RRSensorMode_flg
  bus_selector18 : BusSelector  OutputSignals=VOUTP_S1WheelDebugALTU_pct
  bus_selector19 : BusSelector  OutputSignals=VOUTP_S2WheelDebugALTU_pct
  bus_selector2 : BusSelector  OutputSignals=VOUTP_ID1messageALTU_raw8
  bus_selector20 : BusSelector  OutputSignals=VOUTP_S3WheelDebugALTU_pct
  bus_selector21 : BusSelector  OutputSignals=VOUTP_S4WheelDebugALTU_pct
  bus_selector3 : BusSelector  OutputSignals=VOUTP_S2ID_raw32
  bus_selector4 : BusSelector  OutputSignals=VOUTP_S2L_enum
  bus_selector5 : BusSelector  OutputSignals=VOUTP_ID2messageALTU_raw8
  bus_selector6 : BusSelector  OutputSignals=VOUTP_S3ID_raw32
  bus_selector7 : BusSelector  OutputSignals=VOUTP_S3L_enum
  bus_selector8 : BusSelector  OutputSignals=VOUTP_ID3messageALTU_raw8
  bus_selector9 : BusSelector  OutputSignals=VOUTP_S4ID_raw32
  FD5_Debug1 : Outport
  wires:
  BSCP_outputs/1 -> [BSCP_outputs]
  BOUTP_outputs/1 -> [BOUTP_outputs]
  [CAN5_ID1_ALTU] -> bus_creator/1  "CAN5_ID1_ALTU"
  [CAN5_ID1_Loc_ALTU] -> bus_creator/2  "CAN5_ID1_Loc_ALTU"
  [CAN5_ID1_message_ALTU] -> bus_creator/3  "CAN5_ID1_message_ALTU"
  [CAN5_ID2_ALTU] -> bus_creator/4  "CAN5_ID2_ALTU"
  [CAN5_ID2_Loc_ALTU] -> bus_creator/5  "CAN5_ID2_Loc_ALTU"
  [CAN5_ID2_message_ALTU] -> bus_creator/6  "CAN5_ID2_message_ALTU"
  [CAN5_ID3_ALTU] -> bus_creator/7  "CAN5_ID3_ALTU"
  [CAN5_ID3_Loc_ALTU] -> bus_creator/8  "CAN5_ID3_Loc_ALTU"
  [CAN5_ID3_message_ALTU] -> bus_creator/9  "CAN5_ID3_message_ALTU"
  [CAN5_ID4_ALTU] -> bus_creator/10  "CAN5_ID4_ALTU"
  [CAN5_ID4_Loc_ALTU] -> bus_creator/11  "CAN5_ID4_Loc_ALTU"
  [CAN5_ID4_message_ALTU] -> bus_creator/12  "CAN5_ID4_message_ALTU"
  [CAN5_IDin_ALTU] -> bus_creator/13  "CAN5_IDin_ALTU"
  [CAN5_LFSensorMode] -> bus_creator/14  "CAN5_LFSensorMode"
  [CAN5_LRSensorMode] -> bus_creator/15  "CAN5_LRSensorMode"
  [CAN5_RFSensorMode] -> bus_creator/16  "CAN5_RFSensorMode"
  [CAN5_RF_FAT_ALTU] -> bus_creator/17  "CAN5_RF_FAT_ALTU"
  [CAN5_RRSensorMode] -> bus_creator/18  "CAN5_RRSensorMode"
  [CAN5_S1WheelDebug_ALTU] -> bus_creator/19  "CAN5_S1WheelDebug_ALTU"
  [CAN5_S2WheelDebug_ALTU] -> bus_creator/20  "CAN5_S2WheelDebug_ALTU"
  [CAN5_S3WheelDebug_ALTU] -> bus_creator/21  "CAN5_S3WheelDebug_ALTU"
  [CAN5_S4WheelDebug_ALTU] -> bus_creator/22  "CAN5_S4WheelDebug_ALTU"
  bus_creator/1 -> FD5_Debug1/1
  ID1ALTU/1(CAN5_ID1_ALTU) -> [CAN5_ID1_ALTU]
  ID1LocALTU/1(CAN5_ID1_Loc_ALTU) -> [CAN5_ID1_Loc_ALTU]
  ID1messageALTU/1(CAN5_ID1_message_ALTU) -> [CAN5_ID1_message_ALTU]
  ID2ALTU/1(CAN5_ID2_ALTU) -> [CAN5_ID2_ALTU]
  ID2LocALTU/1(CAN5_ID2_Loc_ALTU) -> [CAN5_ID2_Loc_ALTU]
  ID2messageALTU/1(CAN5_ID2_message_ALTU) -> [CAN5_ID2_message_ALTU]
  ID3ALTU/1(CAN5_ID3_ALTU) -> [CAN5_ID3_ALTU]
  ID3LocALTU/1(CAN5_ID3_Loc_ALTU) -> [CAN5_ID3_Loc_ALTU]
  ID3messageALTU/1(CAN5_ID3_message_ALTU) -> [CAN5_ID3_message_ALTU]
  ID4ALTU/1(CAN5_ID4_ALTU) -> [CAN5_ID4_ALTU]
  ID4LocALTU/1(CAN5_ID4_Loc_ALTU) -> [CAN5_ID4_Loc_ALTU]
  ID4messageALTU/1(CAN5_ID4_message_ALTU) -> [CAN5_ID4_message_ALTU]
  IDinALTU/1(CAN5_IDin_ALTU) -> [CAN5_IDin_ALTU]
  LFSensorMode/1(CAN5_LFSensorMode) -> [CAN5_LFSensorMode]
  LRSensorMode/1(CAN5_LRSensorMode) -> [CAN5_LRSensorMode]
  RFSensorMode/1(CAN5_RFSensorMode) -> [CAN5_RFSensorMode]
  RFFATALTU/1(CAN5_RF_FAT_ALTU) -> [CAN5_RF_FAT_ALTU]
  RRSensorMode/1(CAN5_RRSensorMode) -> [CAN5_RRSensorMode]
  S1WheelDebugALTU/1(CAN5_S1WheelDebug_ALTU) -> [CAN5_S1WheelDebug_ALTU]
  S2WheelDebugALTU/1(CAN5_S2WheelDebug_ALTU) -> [CAN5_S2WheelDebug_ALTU]
  S3WheelDebugALTU/1(CAN5_S3WheelDebug_ALTU) -> [CAN5_S3WheelDebug_ALTU]
  S4WheelDebugALTU/1(CAN5_S4WheelDebug_ALTU) -> [CAN5_S4WheelDebug_ALTU]
  bus_selector/1 -> ID1ALTU/1(ID1ALTU)  "<VOUTP_S1ID_raw32>"
  [BOUTP_outputs] -> bus_selector/1
  bus_selector1/1 -> ID1LocALTU/1(ID1LocALTU)  "<VOUTP_S1L_enum>"
  [BOUTP_outputs] -> bus_selector1/1
  bus_selector2/1 -> ID1messageALTU/1(ID1messageALTU)  "<VOUTP_ID1messageALTU_raw8>"
  [BOUTP_outputs] -> bus_selector2/1
  bus_selector3/1 -> ID2ALTU/1(ID2ALTU)  "<VOUTP_S2ID_raw32>"
  [BOUTP_outputs] -> bus_selector3/1
  bus_selector4/1 -> ID2LocALTU/1(ID2LocALTU)  "<VOUTP_S2L_enum>"
  [BOUTP_outputs] -> bus_selector4/1
  bus_selector5/1 -> ID2messageALTU/1(ID2messageALTU)  "<VOUTP_ID2messageALTU_raw8>"
  [BOUTP_outputs] -> bus_selector5/1
  bus_selector6/1 -> ID3ALTU/1(ID3ALTU)  "<VOUTP_S3ID_raw32>"
  [BOUTP_outputs] -> bus_selector6/1
  bus_selector7/1 -> ID3LocALTU/1(ID3LocALTU)  "<VOUTP_S3L_enum>"
  [BOUTP_outputs] -> bus_selector7/1
  bus_selector8/1 -> ID3messageALTU/1(ID3messageALTU)  "<VOUTP_ID3messageALTU_raw8>"
  [BOUTP_outputs] -> bus_selector8/1
  bus_selector9/1 -> ID4ALTU/1(ID4ALTU)  "<VOUTP_S4ID_raw32>"
  [BOUTP_outputs] -> bus_selector9/1
  bus_selector10/1 -> ID4LocALTU/1(ID4LocALTU)  "<VOUTP_S4L_enum>"
  [BOUTP_outputs] -> bus_selector10/1
  bus_selector11/1 -> ID4messageALTU/1(ID4messageALTU)  "<VOUTP_ID4messageALTU_raw8>"
  [BOUTP_outputs] -> bus_selector11/1
  bus_selector12/1 -> IDinALTU/1(IDinALTU)  "<VOUTP_IDin_raw32>"
  [BOUTP_outputs] -> bus_selector12/1
  bus_selector13/1 -> LFSensorMode/1(LFSensorMode)  "<VOUTP_LFSensorMode_flg>"
  [BOUTP_outputs] -> bus_selector13/1
  bus_selector14/1 -> LRSensorMode/1(LRSensorMode)  "<VOUTP_LRSensorMode_flg>"
  [BOUTP_outputs] -> bus_selector14/1
  bus_selector15/1 -> RFSensorMode/1(RFSensorMode)  "<VOUTP_RFSensorMode_flg>"
  [BOUTP_outputs] -> bus_selector15/1
  bus_selector16/1 -> RFFATALTU/1(RFFATALTU)  "<VOUTP_FAT_flg>"
  [BOUTP_outputs] -> bus_selector16/1
  bus_selector17/1 -> RRSensorMode/1(RRSensorMode)  "<VOUTP_RRSensorMode_flg>"
  [BOUTP_outputs] -> bus_selector17/1
  bus_selector18/1 -> S1WheelDebugALTU/1(S1WheelDebugALTU)  "<VOUTP_S1WheelDebugALTU_pct>"
  [BOUTP_outputs] -> bus_selector18/1
  bus_selector19/1 -> S2WheelDebugALTU/1(S2WheelDebugALTU)  "<VOUTP_S2WheelDebugALTU_pct>"
  [BOUTP_outputs] -> bus_selector19/1
  bus_selector20/1 -> S3WheelDebugALTU/1(S3WheelDebugALTU)  "<VOUTP_S3WheelDebugALTU_pct>"
  [BOUTP_outputs] -> bus_selector20/1
  bus_selector21/1 -> S4WheelDebugALTU/1(S4WheelDebugALTU)  "<VOUTP_S4WheelDebugALTU_pct>"
  [BOUTP_outputs] -> bus_selector21/1
